simulink model "Computed_Pos_Pos_Force"  (R2023b)
settings: Solver=VariableStepAuto  StartTime=0.0  StopTime=10.0  RelTol=1e-3
settings Model: Creator=91996  LastModifiedBy=91996

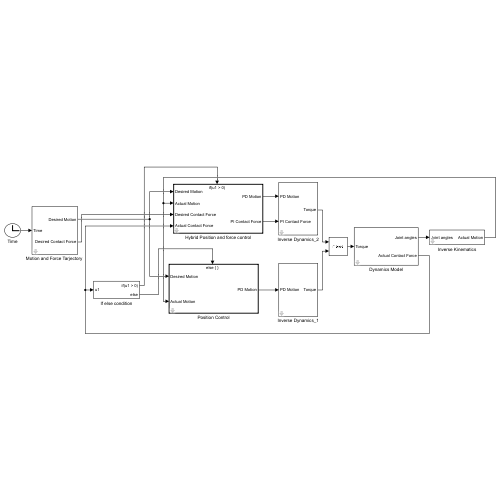
[thumbnail: Simulink's stored preview of the top-level diagram]
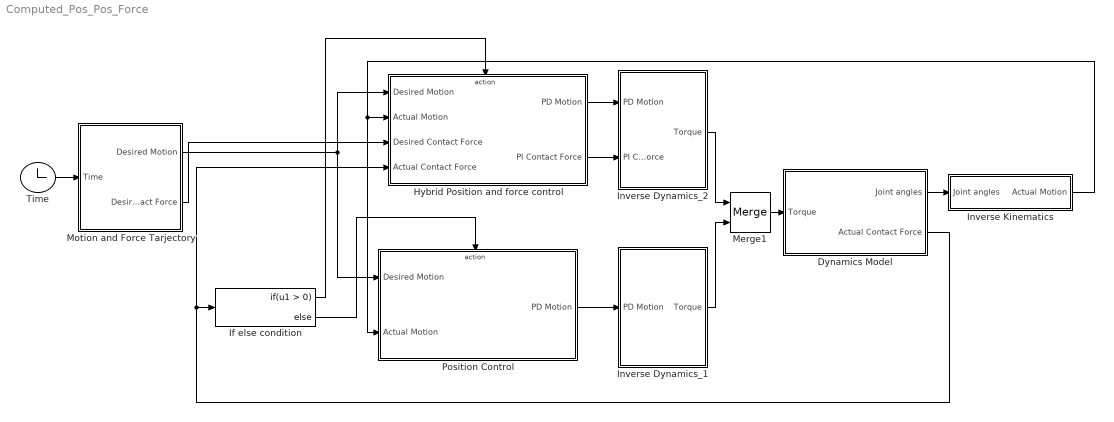
== system Computed_Pos_Pos_Force ==
  Dynamics Model : Subsystem
      mask DialogControl C Prompt: Parameters
  Hybrid Position and force control : Subsystem
      mask DialogControl A Prompt: Parameters
  If else condition : If
  Inverse Dynamics_1 : Subsystem
      mask DialogControl B Prompt: Parameters
  Inverse Dynamics_2 : Subsystem
      mask DialogControl B Prompt: Parameters
  Inverse Kinematics : Subsystem
      mask DialogControl Kinematics Prompt: Parameters
  Merge1 : Merge
  "Motion and Force Tarjectory " : Subsystem
      mask DialogControl E Prompt: Parameters
  Position Control : Subsystem
      mask DialogControl A Prompt: Parameters
  Time : Clock
  wires:
  "Motion and Force Tarjectory "/1(Desired Motion) -> Position Control/1(Desired Motion), Hybrid Position and force control/1(Desired Motion)
  Hybrid Position and force control/1(PD Motion) -> Inverse Dynamics_2/1(PD Motion)
  Time/1 -> "Motion and Force Tarjectory "/1(Time)
  Inverse Kinematics/1(Actual Motion) -> Position Control/2(Actual Motion), Hybrid Position and force control/2(Actual Motion)
  Dynamics Model/1(Joint angles) -> Inverse Kinematics/1(Joint angles)
  "Motion and Force Tarjectory "/2(Desired Contact Force) -> Hybrid Position and force control/3(Desired Contact Force)
  Dynamics Model/2(Actual Contact Force) -> If else condition/1, Hybrid Position and force control/4(Actual Contact Force)
  Hybrid Position and force control/2(PI Contact Force) -> Inverse Dynamics_2/2(PI Contact Force)
  If else condition/2 -> Position Control/Action
  If else condition/1 -> Hybrid Position and force control/Action
  Position Control/1(PD Motion) -> Inverse Dynamics_1/1(PD Motion)
  Merge1/1 -> Dynamics Model/1(Torque)
  Inverse Dynamics_2/1(Torque) -> Merge1/1
  Inverse Dynamics_1/1(Torque) -> Merge1/2

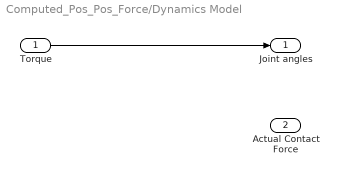
== system Computed_Pos_Pos_Force/Dynamics Model ==
  Torque : Inport
  Joint angles : Outport
  Actual Contact Force : Outport  Port=2
  wires:
  Torque/1 -> Joint angles/1

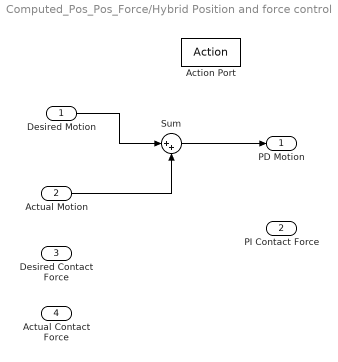
== system Computed_Pos_Pos_Force/Hybrid Position and force control ==
  Desired Motion : Inport
  Actual Motion : Inport  Port=2
  Desired Contact Force : Inport  Port=3
  Actual Contact Force : Inport  Port=4
  Action Port : ActionPort  ActionPortLabel=if(u1 > 0)
  Sum : Sum  Inputs=|++
  PD Motion : Outport
  PI Contact Force : Outport  Port=2
  wires:
  Desired Motion/1 -> Sum/1
  Actual Motion/1 -> Sum/2
  Sum/1 -> PD Motion/1

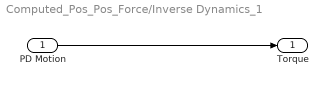
== system Computed_Pos_Pos_Force/Inverse Dynamics_1 ==
  PD Motion : Inport
  Torque : Outport
  wires:
  PD Motion/1 -> Torque/1

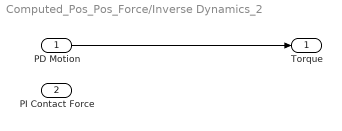
== system Computed_Pos_Pos_Force/Inverse Dynamics_2 ==
  PD Motion : Inport
  PI Contact Force : Inport  Port=2
  Torque : Outport
  wires:
  PD Motion/1 -> Torque/1

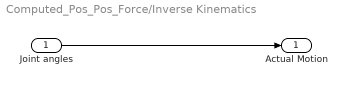
== system Computed_Pos_Pos_Force/Inverse Kinematics ==
  Joint angles : Inport
  Actual Motion : Outport
  wires:
  Joint angles/1 -> Actual Motion/1

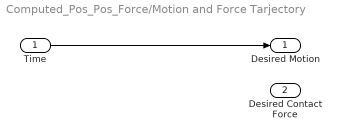
== system Computed_Pos_Pos_Force/Motion and Force Tarjectory  ==
  Time : Inport
  Desired Motion : Outport
  Desired Contact Force : Outport  Port=2
  wires:
  Time/1 -> Desired Motion/1

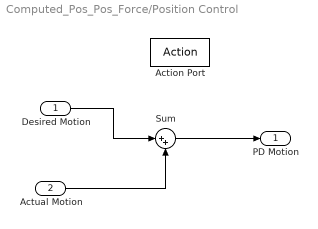
== system Computed_Pos_Pos_Force/Position Control ==
  Desired Motion : Inport
  Actual Motion : Inport  Port=2
  Action Port : ActionPort  ActionPortLabel=else
  Sum : Sum  Inputs=|++
  PD Motion : Outport
  wires:
  Desired Motion/1 -> Sum/1
  Actual Motion/1 -> Sum/2
  Sum/1 -> PD Motion/1
